simulink model "hev_p2_model"  (R2026a)
settings: Solver=ode23tb  StopTime=1800  RelTol=1e-4  AbsTol=1e-5
undefined symbols (not defined in the file): hev
settings Model: Creator=devvr  LastModifiedBy=devvr

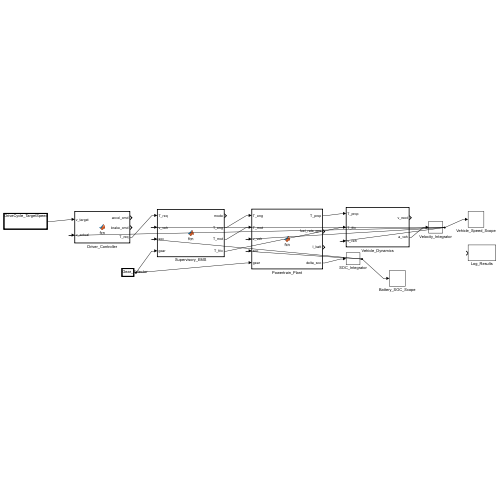
[thumbnail: Simulink's stored preview of the top-level diagram]
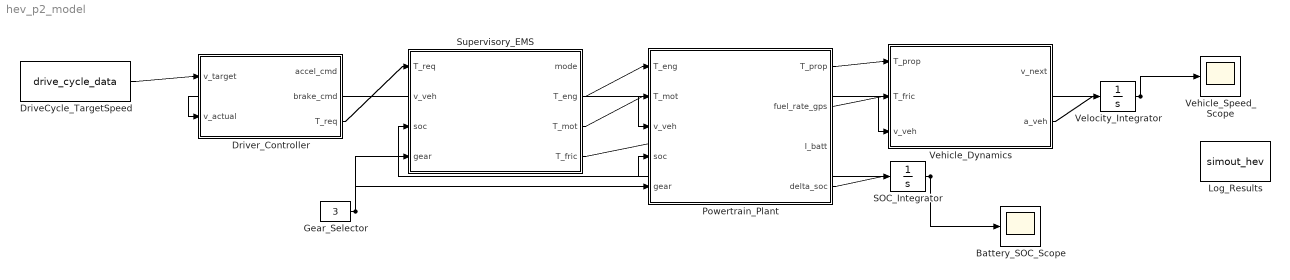
== system hev_p2_model ==
  Battery_SOC_Scope : Scope
  DriveCycle_TargetSpeed : FromWorkspace  VariableName=drive_cycle_data
  Driver_Controller : MATLAB Function  TreatAsAtomicUnit=on
  Gear_Selector : Constant  Value=3
  Log_Results : ToWorkspace  VariableName=simout_hev  SaveFormat=Timeseries  SampleTime=-1
  Powertrain_Plant : MATLAB Function  TreatAsAtomicUnit=on
  SOC_Integrator : Integrator  InitialCondition=hev.ems.soc_target
  Supervisory_EMS : MATLAB Function  TreatAsAtomicUnit=on
  Vehicle_Dynamics : MATLAB Function  TreatAsAtomicUnit=on
  Vehicle_Speed_Scope : Scope
  Velocity_Integrator : Integrator  InitialCondition=0.0
  wires:
  DriveCycle_TargetSpeed/1 -> Driver_Controller/1(v_target)
  Velocity_Integrator/1 -> Driver_Controller/2(v_actual), Supervisory_EMS/2(v_veh), Powertrain_Plant/3(v_veh), Vehicle_Dynamics/3(v_veh), Vehicle_Speed_Scope/1
  Driver_Controller/3(T_req) -> Supervisory_EMS/1(T_req)
  SOC_Integrator/1 -> Supervisory_EMS/3(soc), Powertrain_Plant/4(soc), Battery_SOC_Scope/1
  Gear_Selector/1 -> Supervisory_EMS/4(gear), Powertrain_Plant/5(gear)
  Supervisory_EMS/2(T_eng) -> Powertrain_Plant/1(T_eng)
  Supervisory_EMS/3(T_mot) -> Powertrain_Plant/2(T_mot)
  Powertrain_Plant/4(delta_soc) -> SOC_Integrator/1
  Powertrain_Plant/1(T_prop) -> Vehicle_Dynamics/1(T_prop)
  Supervisory_EMS/4(T_fric) -> Vehicle_Dynamics/2(T_fric)
  Vehicle_Dynamics/2(a_veh) -> Velocity_Integrator/1

== matlab function hev_p2_model/Supervisory_EMS ==
  data: T_req input; mode output; v_veh input; soc input; gear input; T_eng output; T_mot output; T_fric output
function [mode, T_eng, T_mot, T_fric] = Supervisory_EMS(T_req, v_veh, soc, gear)
% Supervisory Energy Management Strategy
v_kmh = v_veh * 3.6;
if T_req < 0
    mode = 5; % Regen Braking
    T_eng = 0;
    if soc < 0.80
        T_mot = max(T_req * 0.80, -170.0);
    else
        T_mot = 0.0;
    end
    T_fric = T_req - T_mot;
elseif T_req == 0
    mode = 1;
    T_eng = 0;
    T_mot = 0;
    T_fric = 0;
else
    T_fric = 0;
    if (v_kmh < 45.0) && (soc > 0.35) && (T_req <= 120.0)
        mode = 1; % Pure EV
        T_eng = 0;
        T_mot = T_req;
    elseif (soc < 0.45) && (T_req < 140.0)
        mode = 4; % Charge / Load shift
        T_eng = 140.0;
        T_mot = T_req - 140.0;
    elseif T_req > 200.0
        mode = 3; % Hybrid Boost
        T_eng = min(T_req, 230.0);
        T_mot = min(T_req - T_eng, 120.0);
    else
        mode = 2; % Engine Only
        T_eng = T_req;
        T_mot = 0;
    end
end

== matlab function hev_p2_model/Driver_Controller ==
  data: v_target input; accel_cmd output; v_actual input; brake_cmd output; T_req output
function [accel_cmd, brake_cmd, T_req] = Driver_Controller(v_target, v_actual)
% Longitudinal Driver PI Controller
persistent int_err;
if isempty(int_err)
    int_err = 0;
end
dt = 0.1;
err = v_target - v_actual;
int_err = int_err + err * dt;
int_err = max(min(int_err, 20.0), -20.0);
Kp = 150.0;
Ki = 12.0;
control_effort = Kp * err + Ki * int_err;
if control_effort >= 0
    accel_cmd = min(control_effort / 200.0, 1.0);
    brake_cmd = 0.0;
    T_req = accel_cmd * 350.0;
else
    accel_cmd = 0.0;
    brake_cmd = min(abs(control_effort) / 200.0, 1.0);
    T_req = -brake_cmd * 400.0;
end

== matlab function hev_p2_model/Powertrain_Plant ==
  data: T_eng input; T_prop output; T_mot input; v_veh input; soc input; gear input; fuel_rate_gps output; I_batt output; delta_soc output
function [T_prop, fuel_rate_gps, I_batt, delta_soc] = Powertrain_Plant(T_eng, T_mot, v_veh, soc, gear)
% Powertrain Plant: Engine, Motor & Battery Model
r_w = 0.315;
diff_ratio = 3.94;
gear_ratios = [3.82, 2.20, 1.45, 1.05, 0.82, 0.68];
g_idx = max(1, min(6, round(gear)));
gr = gear_ratios(g_idx);
total_ratio = gr * diff_ratio;
w_wheel = v_veh / r_w;
w_trans = max(w_wheel * total_ratio, 83.77); % Min 800 RPM in rad/s
T_prop = (T_eng + T_mot) * total_ratio * 0.96;
P_eng_kW = max(0.0, T_eng * w_trans / 1000.0);
if P_eng_kW > 0.1
    bsfc = 240.0; % Approximate mid-range BSFC in g/kWh
    fuel_rate_gps = (P_eng_kW * bsfc) / 3600.0;
else
    fuel_rate_gps = 0.0;
end
P_elec_W = T_mot * w_trans;
if P_elec_W >= 0
    P_batt_W = P_elec_W / 0.92; % Inverter/motor motoring efficiency
else
    P_batt_W = P_elec_W * 0.88; % Regen generation efficiency
end
V_nom = 355.2;
I_batt = P_batt_W / V_nom;
Q_batt = 4.5 * 3600.0; % Amp-seconds
delta_soc = -I_batt / Q_batt;

== matlab function hev_p2_model/Vehicle_Dynamics ==
  data: T_prop input; v_next output; T_fric input; v_veh input; a_veh output
function [v_next, a_veh] = Vehicle_Dynamics(T_prop, T_fric, v_veh)
% Longitudinal Vehicle Body Equations of Motion
mass_eff = 1480.0 * 1.05;
r_w = 0.315;
rho = 1.205;
Cd = 0.28;
Af = 2.22;
cr = 0.011;
g = 9.81;
F_tractive = T_prop / r_w;
F_aero = 0.5 * rho * Cd * Af * (v_veh^2);
if v_veh > 0.05
    F_roll = cr * 1480.0 * g;
else
    F_roll = 0.0;
end
F_fric_brake = (T_fric / r_w);
F_net = F_tractive - F_aero - F_roll + F_fric_brake;
a_veh = F_net / mass_eff;
v_next = max(0.0, v_veh + a_veh * 0.1);
